simulink model "difference_filter"  (R2019a)
settings: Solver=VariableStepAuto  StartTime=0.0  StopTime=0.02  RelTol=1e-3
libraries: dsparch4 x4, commrandsrc3 x1
settings Model: Creator=Birkan  LastModifiedBy=Birkan

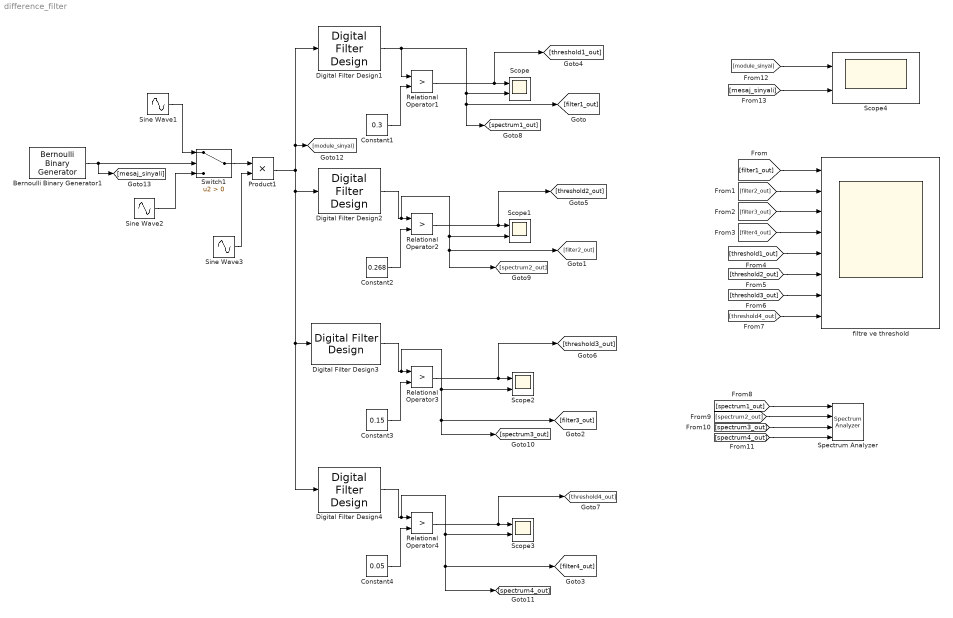
== system difference_filter ==
  Bernoulli Binary Generator1 : commrandsrc3/Bernoulli Binary Generator  ProbabilityOfZero=0.5  SeedSource=Auto  Seed=0  SampleTime=0.003  SamplesPerFrame=1  OutputDataType=double  SimulateUsing=Interpreted execution
      settings: SourceProductName=Communications Toolbox
  Constant1 : Constant  Value=0.3
  Constant2 : Constant  Value=0.268
  Constant3 : Constant  Value=0.15
  Constant4 : Constant  Value=0.05
  Digital Filter Design{1..4} (4 alike) : dsparch4/Digital Filter Design  mwdsp_browser_bugfix_var=off
  Product1 : Product
  Relational Operator{1..4} (4 alike) : RelationalOperator  Operator=>  OutDataTypeStr=boolean  RndMeth=Simplest
  Scope{,1..4} (5 alike) : Scope  NumInputPorts=2
  Sine Wave1 : Sin  Frequency=20000*pi  SampleTime=1/1000000
  Sine Wave2 : Sin  Amplitude=0.14  Frequency=20000*pi  SampleTime=1/1000000
  Sine Wave3 : Sin  Frequency=20000*pi  SampleTime=1/1000000
  Spectrum Analyzer : SpectrumAnalyzer  NumInputPorts=4
  Switch1 : Switch  Criteria=u2 > Threshold
  "filtre ve threshold " : Scope  NumInputPorts=8
  wires:
  Sine Wave3/1 -> Product1/2
  Digital Filter Design1/1 -> [filter1_out], [spectrum1_out], Scope/2, Relational Operator1/1
  Product1/1 -> Digital Filter Design1/1, [module_sinyal], Digital Filter Design4/1, Digital Filter Design3/1, Digital Filter Design2/1
  Switch1/1 -> Product1/1
  Constant1/1 -> Relational Operator1/2
  Sine Wave2/1 -> Switch1/3
  Sine Wave1/1 -> Switch1/1
  Relational Operator1/1 -> [threshold1_out], Scope/1
  Constant2/1 -> Relational Operator2/2
  Digital Filter Design2/1 -> Scope1/2, [filter2_out], [spectrum2_out], Relational Operator2/1
  Relational Operator2/1 -> [threshold2_out], Scope1/1
  Constant3/1 -> Relational Operator3/2
  Digital Filter Design3/1 -> Scope2/2, [spectrum3_out], [filter3_out], Relational Operator3/1
  Relational Operator3/1 -> [threshold3_out], Scope2/1
  Constant4/1 -> Relational Operator4/2
  Digital Filter Design4/1 -> Scope3/2, [filter4_out], [spectrum4_out], Relational Operator4/1
  Relational Operator4/1 -> [threshold4_out], Scope3/1
  [filter1_out] -> "filtre ve threshold "/1
  [filter2_out] -> "filtre ve threshold "/2
  [filter3_out] -> "filtre ve threshold "/3
  [filter4_out] -> "filtre ve threshold "/4
  [threshold1_out] -> "filtre ve threshold "/5
  [threshold2_out] -> "filtre ve threshold "/6
  [threshold3_out] -> "filtre ve threshold "/7
  [threshold4_out] -> "filtre ve threshold "/8
  [spectrum1_out] -> Spectrum Analyzer/1
  [spectrum2_out] -> Spectrum Analyzer/2
  [spectrum3_out] -> Spectrum Analyzer/3
  [spectrum4_out] -> Spectrum Analyzer/4
  [module_sinyal] -> Scope4/1
  Bernoulli Binary Generator1/1 -> [mesaj_sinyali], Switch1/2
  [mesaj_sinyali] -> Scope4/2
